simulink library "InLineRmsBtc"  (R2022b)
settings: Solver=VariableStepAuto  StartTime=0.0  StopTime=10.0  RelTol=1e-3
undefined symbols (not defined in the file or in its folder): Row
libraries: TuneVar x5, RTC x2, FeaturePath x1, HandyTextFile x1, AudioStats x1, TOP x1
settings Model: Creator=kl13806  LastModifiedBy=kl13806
settings SolverCC: AlgebraicLoopSolver=TrustRegion
settings DebuggingCC: UnconnectedInputMsg=warning  UnconnectedOutputMsg=warning  UnconnectedLineMsg=warning  SFMachineParentedDataDiag=warning
settings ModelReferenceCC: EnableRefExpFcnMdlSchedulingChecks=on
settings RTWCC: DLArmComputeVersion=19.05

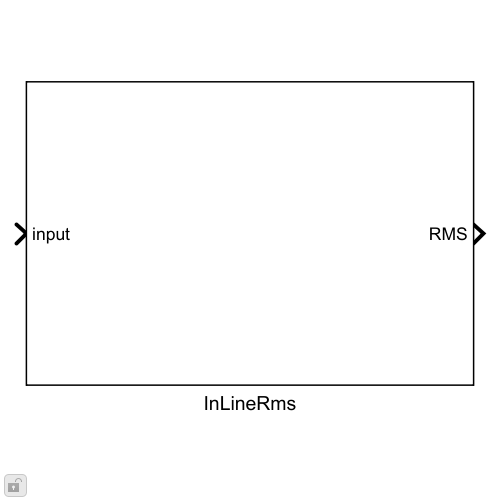
[thumbnail: Simulink's stored preview of the top-level diagram]
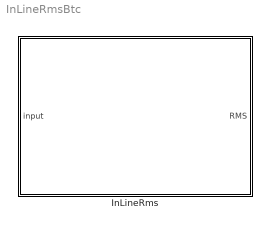
== system InLineRmsBtc ==
  InLineRms : Subsystem  mask(Blocklib InLineRms){Config=[], FeatureName=RMS}
      mask prompts: Config "InLineRmsConfig"; FeatureName "Feature path name:"
      mask help: RMS block calculates RMS/MS values for multiple channels individually
      mask init:
      | blkh=gcbh;
      | Config=BTConfig.Assert(blkh,Config);
      | Config.Validate();
      | BTConfig.InitSetFeatureIfPresent(blkh,'FeatureName');
      mask Callback Config: BTConfig.CallbackHideIfPresent(gcbh,{'FeatureName'});
      mask TypeOptions FeatureName: FeaturePath/FeatureName

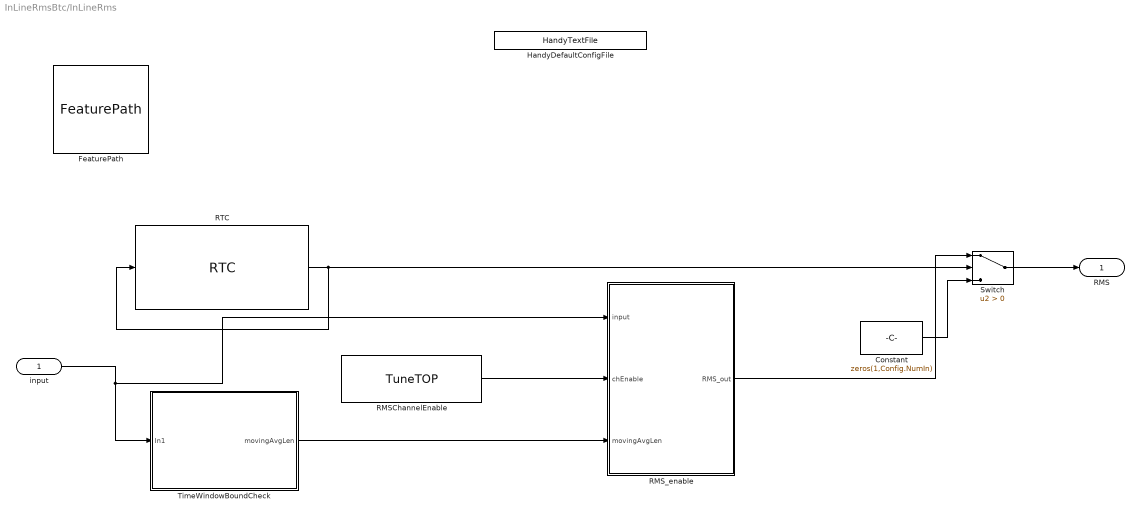
== system InLineRmsBtc/InLineRms ==
  input : Inport
  Constant : Constant  Value=zeros(1,Config.NumIn)  VectorParams1D=off  OutDataTypeStr=single
  FeaturePath : FeaturePath/FeaturePath  FeatureName=RMS  IsGroup=off  GroupNumber=-1  IsModule=off  TriggerInit=[-295 179 -180 286]
      settings: SourceProductName=Bose Talaria
  HandyDefaultConfigFile : HandyTextFile/HandyTextFile  TemplateSource=Config  FileSuffix=Init  OpenDialogOnLoad=off  UseThisBlockName=off  AddGrandParentNamePrefix=off  TheDefaultText=|  ShowInLibBrowser=on
      | % $(FILENAME) Setup model parameters for each "Init" callback (e.g. update diagram)
      | sample_rate_in_hertz = 44100;
      | frame_size = 32;
      | sysin_channel_count = 2;
      settings: SourceProductName=Bose Talaria
  RMSChannelEnable : TuneVar/TuneTOP  TriggerInit=[55 532 225 588]  TopName=ChannelEnable  TuneName=ChannelEnable  DataType=single  TunabilityNumber=1  MinValue=[]  MaxValue=[]  BankNumber=0  PreOverlay=false  PostOverlay=false  UseSameName=on  MaskValue=Config.DefaultChannelEnable
      settings: SourceProductName=Bose Talaria
  RMS_enable : Subsystem  TreatAsAtomicUnit=on
  RTC : RTC/RTC  REQ_Priority=RTC_Mask.NormalPriority  RequestAtInit=off  EnableRequest=off  REQElemName1=enable  REQElemType1=uint32  REQElemWidth1=1  REQElemInitial1=Config.InitialEnable  REQElemType2=uint32  REQElemWidth2=1  REQElemInitial2=[]  REQElemType3=uint32  REQElemWidth3=1  REQElemInitial3=[]  REQElemType4=uint32  REQElemWidth4=1  REQElemInitial4=[]  REQElemType5=uint32  REQElemWidth5=1  REQElemInitial5=[]  REQElemType6=uint32  REQElemWidth6=1  REQElemInitial6=[]  REQElemType7=uint32  REQElemWidth7=1  REQElemInitial7=[]  REQElemType8=uint32  REQElemWidth8=1  REQElemInitial8=[]  REQElemType9=uint32  REQElemWidth9=1  REQElemInitial9=[]  REQElemType10=uint32  REQElemWidth10=1  REQElemInitial10=[]  EnableResponse=on  EnableRSP_StatusIn=off  RSPElemName1=EnableResponsePayload  RSPElemType1=uint32  RSPElemWidth1=1  RSPElemType2=uint32  RSPElemWidth2=1  RSPElemType3=uint32  RSPElemWidth3=1  RSPElemType4=uint32  RSPElemWidth4=1  RSPElemType5=uint32  RSPElemWidth5=1  RSPElemType6=uint32  RSPElemWidth6=1  RSPElemType7=uint32  RSPElemWidth7=1  RSPElemType8=uint32  RSPElemWidth8=1  RSPElemType9=uint32  RSPElemWidth9=1  RSPElemType10=uint32  RSPElemWidth10=1  EnableNotification=off  EnableNTF_PrepTrig=off  NTFElemType1=uint32  NTFElemWidth1=1  NTFElemType2=uint32  NTFElemWidth2=1  NTFElemType3=uint32  NTFElemWidth3=1  NTFElemType4=uint32  NTFElemWidth4=1  NTFElemType5=uint32  NTFElemWidth5=1  NTFElemType6=uint32  NTFElemWidth6=1  NTFElemType7=uint32  NTFElemWidth7=1  NTFElemType8=uint32  NTFElemWidth8=1  NTFElemType9=uint32  NTFElemWidth9=1  NTFElemType10=uint32  NTFElemWidth10=1  MaskMessageName=Enable
      settings: SourceProductName=Bose Talaria
  Switch : Switch  Criteria=u2 > Threshold  SaturateOnIntegerOverflow=off  InputSameDT=off
  TimeWindowBoundCheck : Subsystem
  RMS : Outport
  wires:
  TimeWindowBoundCheck/1(movingAvgLen) -> RMS_enable/3(movingAvgLen)
  Constant/1 -> Switch/3
  Switch/1 -> RMS/1
  RMS_enable/1(RMS_out) -> Switch/1
  RTC/1 -> RTC/1, Switch/2
  input/1 -> RMS_enable/1(input), TimeWindowBoundCheck/1(In1)
  RMSChannelEnable/1 -> RMS_enable/2(chEnable)

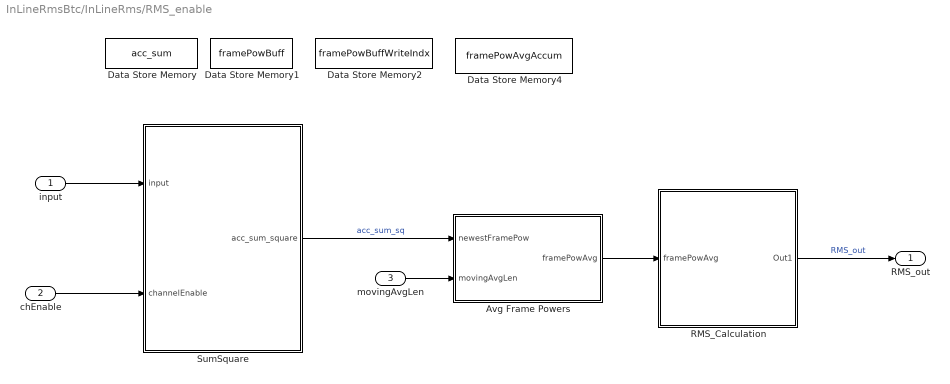
== system InLineRmsBtc/InLineRms/RMS_enable ==
  input : Inport
  chEnable : Inport  Port=2
  movingAvgLen : Inport  Port=3
  Avg Frame Powers : MATLAB Function  TreatAsAtomicUnit=on
  Data Store Memory : DataStoreMemory  DataStoreName=acc_sum  InitialValue=zeros(1,Config.NumIn)  VectorParams1D=off  ShowAdditionalParam=off  OutDataTypeStr=single
  Data Store Memory1 : DataStoreMemory  DataStoreName=framePowBuff  ReadBeforeWriteMsg=warning  WriteAfterWriteMsg=warning  WriteAfterReadMsg=warning  InitialValue=zeros(1512,Config.NumIn)  VectorParams1D=off  ShowAdditionalParam=off  OutDataTypeStr=single
  Data Store Memory2 : DataStoreMemory  DataStoreName=framePowBuffWriteIndx  ReadBeforeWriteMsg=warning  WriteAfterWriteMsg=warning  WriteAfterReadMsg=warning  InitialValue=1  ShowAdditionalParam=off  OutDataTypeStr=single
  Data Store Memory4 : DataStoreMemory  DataStoreName=framePowAvgAccum  ReadBeforeWriteMsg=warning  WriteAfterWriteMsg=warning  WriteAfterReadMsg=warning  InitialValue=zeros(1,Config.NumIn)  VectorParams1D=off  ShowAdditionalParam=off  OutDataTypeStr=single
  RMS_Calculation : Subsystem  TreatAsAtomicUnit=on
  SumSquare : MATLAB Function  TreatAsAtomicUnit=on  mask{numIn=Config.NumIn}
  RMS_out : Outport
  wires:
  movingAvgLen/1 -> Avg Frame Powers/2(movingAvgLen)
  Avg Frame Powers/1(framePowAvg) -> RMS_Calculation/1(framePowAvg)
  SumSquare/1(acc_sum_square) -> Avg Frame Powers/1(newestFramePow)  "acc_sum_sq"
  RMS_Calculation/1(Out1) -> RMS_out/1  "RMS_out"
  input/1 -> SumSquare/1(input)
  chEnable/1 -> SumSquare/2(channelEnable)

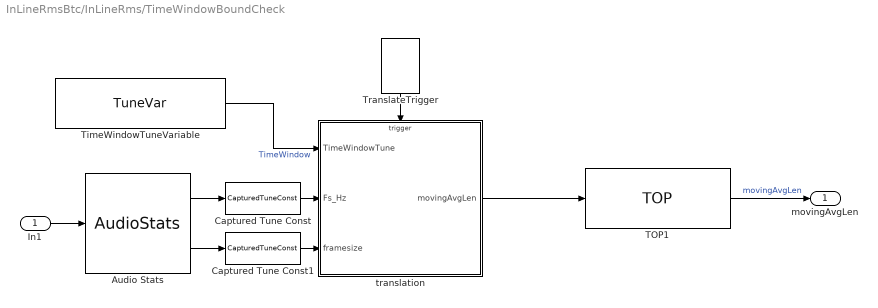
== system InLineRmsBtc/InLineRms/TimeWindowBoundCheck ==
  In1 : Inport
  Audio Stats : AudioStats/AudioStats  DoSampleRate=on  TypeSampleRate=Inherit: auto  DoCallRate=off  TypeCallRate=Inherit: auto  DoFrameSize=on  TypeFrameSize=Inherit: auto  DoChannelCount=off  TypeChannelCount=Inherit: auto  DoTaskRateFactor=off  TypeTaskRateFactor=Inherit: auto  MacroNameRoot=AUDIO  MacroNameRootEval='AUDIO'  IsMacroNameEval=off  MacroSampleRate=off  MacroCallRate=off  MacroFrameSize=off  MacroChannelCount=off  MacroTaskRateFactor=off  MacroTaskId=off  ValidateSampleRate=off  ValueSampleRate=44100  ValidateCallRate=off  ValueCallRate=[]  ValidateFrameSize=off  ValueFrameSize=32  ValidateChannelCount=off  ValueChannelCount=[]  ValidateTaskRateFactor=off  ValueTaskRateFactor=[]
      settings: SourceProductName=Bose Talaria
  Captured Tune Const : TuneVar/CapturedTuneConst  TriggerInit=[185 164 260 196]  Role=Automatic
      settings: SourceProductName=Bose Talaria
  Captured Tune Const1 : TuneVar/CapturedTuneConst  TriggerInit=[185 214 260 246]  Role=Automatic
      settings: SourceProductName=Bose Talaria
  TOP1 : TOP/TOP  TriggerInit=[545 150 690 210]  TopName=movingAvgLen  DataType=uint32  BankNumber=0  PreOverlay=false  PostOverlay=false  Role=Automatic
      settings: SourceProductName=Bose Talaria
  TimeWindowTuneVariable : TuneVar/TuneVar  TuneName=TimeWindow  SpecifyMaxSize=off  VariableDim=1 (Row)  MaxSize=[1 1]  TunabilityNumber=1  MinValue=[]  MaxValue=[]  TriggerInit=[15 60 185 110]  MaskValue=Config.DefaultTimeWindowMs
      settings: SourceProductName=Bose Talaria
  TranslateTrigger : TuneVar/TranslateTrigger  TriggerInit=[341 20 379 75]
      settings: SourceProductName=Bose Talaria
  translation : MATLAB Function  TreatAsAtomicUnit=on  mask{timeWindowBounds=Config.TimeWindowBounds}
  movingAvgLen : Outport
  wires:
  translation/1(movingAvgLen) -> TOP1/1
  TOP1/1 -> movingAvgLen/1  "movingAvgLen"
  TranslateTrigger/1 -> translation/Trigger
  TimeWindowTuneVariable/1 -> translation/1(TimeWindowTune)  "TimeWindow"
  In1/1 -> Audio Stats/1
  Audio Stats/1 -> Captured Tune Const/1
  Audio Stats/2 -> Captured Tune Const1/1
  Captured Tune Const/1 -> translation/2(Fs_Hz)
  Captured Tune Const1/1 -> translation/3(framesize)

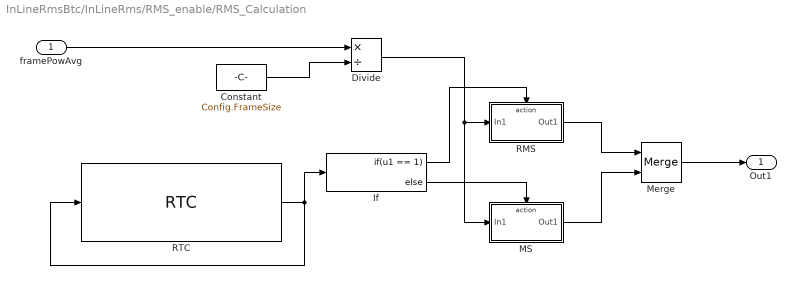
== system InLineRmsBtc/InLineRms/RMS_enable/RMS_Calculation ==
  framePowAvg : Inport
  Constant : Constant  Value=Config.FrameSize  OutDataTypeStr=single
  Divide : Product  Inputs=*/
  If : If  IfExpression=u1 == 1
  MS : Subsystem  TreatAsAtomicUnit=on
  Merge : Merge
  RMS : Subsystem  TreatAsAtomicUnit=on
  RTC : RTC/RTC  REQ_Priority=RTC_Mask.NormalPriority  RequestAtInit=off  EnableRequest=off  REQElemName1=outputRMS  REQElemType1=uint32  REQElemWidth1=1  REQElemInitial1=1  REQElemType2=uint32  REQElemWidth2=1  REQElemInitial2=[]  REQElemType3=uint32  REQElemWidth3=1  REQElemInitial3=[]  REQElemType4=uint32  REQElemWidth4=1  REQElemInitial4=[]  REQElemType5=uint32  REQElemWidth5=1  REQElemInitial5=[]  REQElemType6=uint32  REQElemWidth6=1  REQElemInitial6=[]  REQElemType7=uint32  REQElemWidth7=1  REQElemInitial7=[]  REQElemType8=uint32  REQElemWidth8=1  REQElemInitial8=[]  REQElemType9=uint32  REQElemWidth9=1  REQElemInitial9=[]  REQElemType10=uint32  REQElemWidth10=1  REQElemInitial10=[]  EnableResponse=on  EnableRSP_StatusIn=off  RSPElemName1=ResponsePayload  RSPElemType1=uint32  RSPElemWidth1=1  RSPElemType2=uint32  RSPElemWidth2=1  RSPElemType3=uint32  RSPElemWidth3=1  RSPElemType4=uint32  RSPElemWidth4=1  RSPElemType5=uint32  RSPElemWidth5=1  RSPElemType6=uint32  RSPElemWidth6=1  RSPElemType7=uint32  RSPElemWidth7=1  RSPElemType8=uint32  RSPElemWidth8=1  RSPElemType9=uint32  RSPElemWidth9=1  RSPElemType10=uint32  RSPElemWidth10=1  EnableNotification=off  EnableNTF_PrepTrig=off  NTFElemType1=uint32  NTFElemWidth1=1  NTFElemType2=uint32  NTFElemWidth2=1  NTFElemType3=uint32  NTFElemWidth3=1  NTFElemType4=uint32  NTFElemWidth4=1  NTFElemType5=uint32  NTFElemWidth5=1  NTFElemType6=uint32  NTFElemWidth6=1  NTFElemType7=uint32  NTFElemWidth7=1  NTFElemType8=uint32  NTFElemWidth8=1  NTFElemType9=uint32  NTFElemWidth9=1  NTFElemType10=uint32  NTFElemWidth10=1  MaskMessageName=OutputRMS
      settings: SourceProductName=Bose Talaria
  Out1 : Outport
  wires:
  Constant/1 -> Divide/2
  framePowAvg/1 -> Divide/1
  RTC/1 -> If/1, RTC/1
  If/2 -> MS/Action
  If/1 -> RMS/Action
  Divide/1 -> MS/1(In1), RMS/1(In1)
  RMS/1(Out1) -> Merge/1
  MS/1(Out1) -> Merge/2
  Merge/1 -> Out1/1

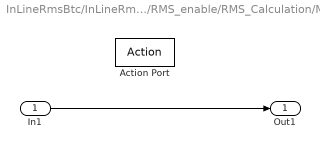
== system InLineRmsBtc/InLineRms/RMS_enable/RMS_Calculation/MS ==
  In1 : Inport
  Action Port : ActionPort
  Out1 : Outport
  wires:
  In1/1 -> Out1/1

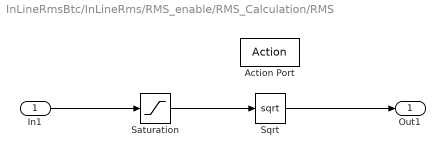
== system InLineRmsBtc/InLineRms/RMS_enable/RMS_Calculation/RMS ==
  In1 : Inport
  Action Port : ActionPort
  Saturation : Saturate  UpperLimit=32767  LowerLimit=0  LinearizeAsGain=off  ZeroCross=off
  Sqrt : Sqrt
  Out1 : Outport
  wires:
  Saturation/1 -> Sqrt/1
  In1/1 -> Saturation/1
  Sqrt/1 -> Out1/1

== matlab function InLineRmsBtc/InLineRms/RMS_enable/Avg Frame Powers ==
  data: newestFramePow input single; framePowAvg output single; framePowBuff data_store_memory; framePowBuffWriteIndx data_store_memory; framePowAvgAccum data_store_memory; movingAvgLen input
function framePowAvg = fcn(newestFramePow, movingAvgLen)
%#codegen
% datastore memory
global framePowBuff;
global framePowBuffWriteIndx;
global framePowAvgAccum;
%
%
buffLen = single(length(framePowBuff));
% Put newest frame power in buffer
framePowBuff(framePowBuffWriteIndx,:) = newestFramePow;
% get read index of old frame power to subtract from running sum
framePowBuffReadIndx = framePowBuffWriteIndx - single(movingAvgLen);
if framePowBuffReadIndx < 1
    framePowBuffReadIndx = framePowBuffReadIndx + buffLen;
end
% add in newest frame power and subtract oldest one
framePowAvgAccum = framePowAvgAccum + newestFramePow;
framePowAvgAccum = framePowAvgAccum - framePowBuff(framePowBuffReadIndx,:);
% increment write index
framePowBuffWriteIndx = framePowBuffWriteIndx + 1;
if framePowBuffWriteIndx > buffLen
    framePowBuffWriteIndx = single(1);
end
% Return newest Avg to output
framePowAvg = framePowAvgAccum/single(movingAvgLen);

== matlab function InLineRmsBtc/InLineRms/RMS_enable/SumSquare ==
  data: acc_sum_square output; input input; acc_sum data_store_memory; channelEnable input; numIn parameter
function acc_sum_square  = sumsquare(input, channelEnable, numIn)
    %#codegen
    % datastore memory to capture the sum of squares value
    global acc_sum;
    
    % Compute sum_of_squares if corresponding channel is enabled(which is a Tune message)
    for ch = 1:numIn
        acc_sum(ch) = 0;
        if(channelEnable(ch) == 1)
            acc_sum(ch) = acc_sum(ch)+ sum(input(:,ch).^2);
        end
    end
    acc_sum_square = acc_sum;

== matlab function InLineRmsBtc/InLineRms/TimeWindowBoundCheck/translation ==
  data: TimeWindowTune input; Fs_Hz input; framesize input; timeWindowBounds parameter; movingAvgLen output
  events: trigger input FUNCTION_CALL_EVENT
function movingAvgLen = fcn(TimeWindowTune, Fs_Hz, framesize, timeWindowBounds)

% datastore memory to capture block size
% TimeWindow is a tune parameter that specifies the duration over which the RMS value should be 
% calculated.  This duration is specified in milli seconds, and is in the range of 1 milli second
% to 1000 milli seconds. If it is configured > 1000 or < 1 then parameter value should be capped
% to '1000' and '1' respectively.

% Warnings were removed since they shouldn't be in blocklib
if TimeWindowTune.Value > timeWindowBounds(2)
    timeWindow_ms = timeWindowBounds(2);
    % TranslateWarning('Time window must be in the ran ge of 1 to 1000 milli seconds, so tuned value is capped in the given range.');
elseif TimeWindowTune.Value < timeWindowBounds(1)
    timeWindow_ms = timeWindowBounds(1);
    % TranslateWarning('Time window must be in the range of 1 to 1000 milli seconds, so tuned value is capped in the given range.');
else
    timeWindow_ms = TimeWindowTune.Value;
end

time_window_secs = timeWindow_ms/1000;
% Ensure that there is at least one frame
movingAvgLen  = max( round((time_window_secs*Fs_Hz) / framesize) ,1);
movingAvgLen = single(movingAvgLen);
